simulink model "Modelo_Tanque_MQR"  (R2022a)
settings: Solver=FixedStepAuto  StartTime=0.0  StopTime=6000  FixedStep=1e-3  RelTol=1e-3
libraries: simulink x1
settings Model: Creator=User  LastModifiedBy=User
settings DebuggingCC: UnconnectedInputMsg=warning  UnconnectedOutputMsg=warning  UnconnectedLineMsg=warning
settings RTWCC: DLArmComputeVersion=19.05

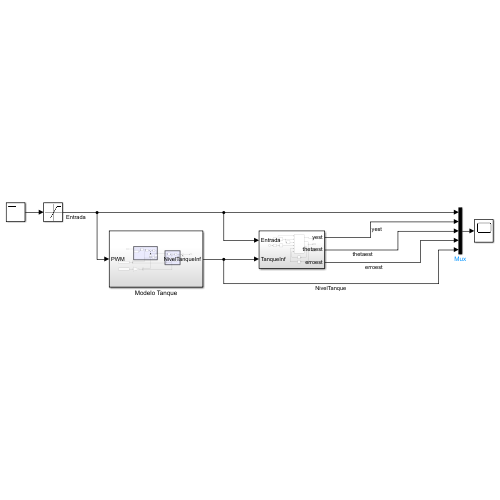
[thumbnail: Simulink's stored preview of the top-level diagram]
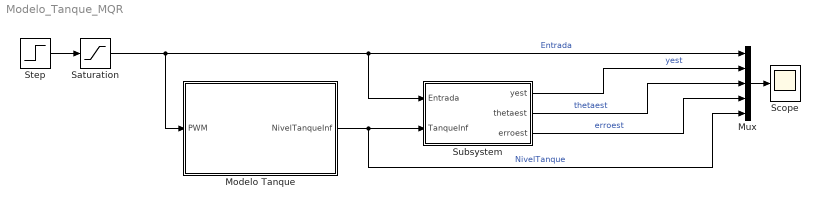
== system Modelo_Tanque_MQR ==
  Modelo Tanque : Subsystem
  Mux : Mux  Inputs=5
  Saturation : Saturate  UpperLimit=1  LowerLimit=0
  Scope : Scope
  Step : Step  Time=3000  Before=0.8  After=0.3  SampleTime=0
  Subsystem : Subsystem
  wires:
  Step/1 -> Saturation/1
  Modelo Tanque/1(NivelTanqueInf) -> Subsystem/2(TanqueInf), Mux/5  "NivelTanque"
  Mux/1 -> Scope/1
  Saturation/1 -> Subsystem/1(Entrada), Mux/1, Modelo Tanque/1(PWM)  "Entrada"
  Subsystem/1(yest) -> Mux/2  "yest"
  Subsystem/2(thetaest) -> Mux/3  "thetaest"
  Subsystem/3(erroest) -> Mux/4  "erroest"

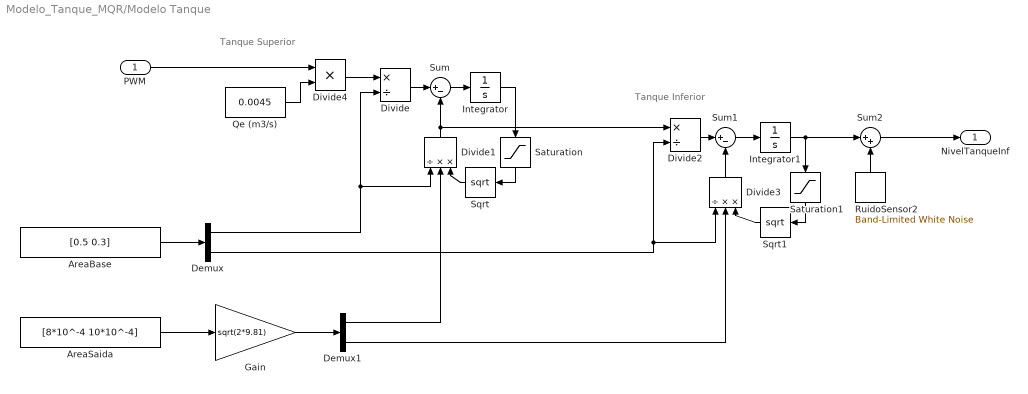
== system Modelo_Tanque_MQR/Modelo Tanque ==
  note: Tanque Inferior
  note: Tanque Superior
  PWM : Inport
  AreaBase : Constant  Value=[0.5 0.3]
  AreaSaida : Constant  Value=[8*10^-4 10*10^-4]
  Demux : Demux  Outputs=2
  Demux1 : Demux  Outputs=2
  Divide : Product  Inputs=*/
  Divide1 : Product  Inputs=/**
  Divide2 : Product  Inputs=*/
  Divide3 : Product  Inputs=/**
  Divide4 : Product  Inputs=**
  Gain : Gain  Gain=sqrt(2*9.81)
  Integrator : Integrator
  Integrator1 : Integrator
  Qe (m3/s) : Constant  Value=0.0045
  RuidoSensor2 : simulink/Sources/Band-Limited White Noise  Cov=[0.00001]  Ts=1  seed=[23341]
  Saturation : Saturate  UpperLimit=inf  LowerLimit=0
  Saturation1 : Saturate  UpperLimit=inf  LowerLimit=0
  Sqrt : Sqrt
  Sqrt1 : Sqrt
  Sum : Sum  Inputs=|+-
  Sum1 : Sum  Inputs=|+-
  Sum2 : Sum  Inputs=|++
  NivelTanqueInf : Outport
  wires:
  AreaSaida/1 -> Gain/1
  AreaBase/1 -> Demux/1
  Gain/1 -> Demux1/1
  Integrator/1 -> Saturation/1
  Demux/1 -> Divide/2, Divide1/1
  Divide/1 -> Sum/1
  Sum/1 -> Integrator/1
  Demux1/1 -> Divide1/2
  Sqrt/1 -> Divide1/3
  Integrator1/1 -> Saturation1/1, Sum2/1
  Demux1/2 -> Divide3/2
  Sqrt1/1 -> Divide3/3
  Divide3/1 -> Sum1/2
  Demux/2 -> Divide3/1, Divide2/2
  Sum1/1 -> Integrator1/1
  Divide2/1 -> Sum1/1
  Sum2/1 -> NivelTanqueInf/1
  RuidoSensor2/1 -> Sum2/2
  Divide1/1 -> Divide2/1, Sum/2
  Saturation/1 -> Sqrt/1
  Saturation1/1 -> Sqrt1/1
  Divide4/1 -> Divide/1
  Qe (m3/s)/1 -> Divide4/2
  PWM/1 -> Divide4/1

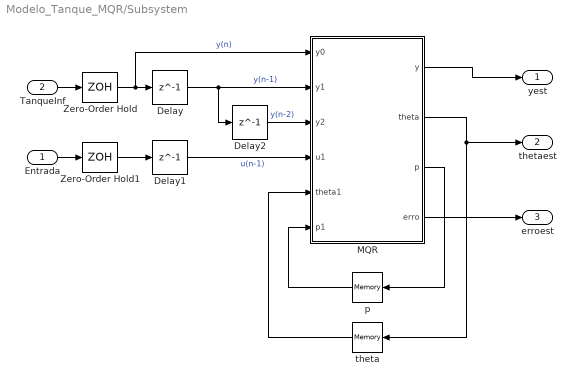
== system Modelo_Tanque_MQR/Subsystem ==
  Entrada : Inport
  TanqueInf : Inport  Port=2
  Delay : Delay  DelayLength=1  InitialCondition=0
  Delay1 : Delay  DelayLength=1  InitialCondition=0
  Delay2 : Delay  DelayLength=1  InitialCondition=0
  MQR : MATLAB Function  TreatAsAtomicUnit=on
  Zero-Order Hold : ZeroOrderHold  SampleTime=10
  Zero-Order Hold1 : ZeroOrderHold  SampleTime=10
  p : Memory  InitialCondition=1000*eye(3)  InheritSampleTime=on
  theta : Memory  InitialCondition=zeros(3,1)  InheritSampleTime=on
  yest : Outport
  thetaest : Outport  Port=2
  erroest : Outport  Port=3
  wires:
  Entrada/1 -> Zero-Order Hold1/1
  TanqueInf/1 -> Zero-Order Hold/1
  MQR/1(y) -> yest/1
  Zero-Order Hold1/1 -> Delay1/1
  Delay1/1 -> MQR/4(u1)  "u(n-1)"
  Delay/1 -> Delay2/1, MQR/2(y1)  "y(n-1)"
  Delay2/1 -> MQR/3(y2)  "y(n-2)"
  MQR/3(p) -> p/1
  MQR/2(theta) -> thetaest/1, theta/1
  theta/1 -> MQR/5(theta1)
  p/1 -> MQR/6(p1)
  Zero-Order Hold/1 -> Delay/1, MQR/1(y0)  "y(n)"
  MQR/4(erro) -> erroest/1

== matlab function Modelo_Tanque_MQR/Subsystem/MQR ==
  data: y0 input; y1 input; y2 input; u1 input; theta1 input; p1 input; y output; theta output; p output; erro output
function [y, theta, p, erro] = fcn(y0, y1, y2, u1, theta1, p1)

lambda1 = 0.99;
lambda2 = 1;

lambda = lambda1/lambda2;

fi = [-y1;...
      -y2;...
       u1];

erro = y0-fi'*theta1;       % Calcula erro de estimação

k = p1*fi/(lambda+fi'*p1*fi);               % Atualiza vetor de ajuste do theta

theta=theta1+k*erro;      % Atualiza o theta

p=(p1-k*fi'*p1)/lambda1;                  % Atualiza matriz de covariância

y = fi'*theta;                 % Calcula a saída a partir dos thetas estimados
